simulink model "PWMverwerking"  (R2018b)
settings: Solver=VariableStepAuto  StartTime=0.0  StopTime=10.0  RelTol=1e-3
undefined symbols (not defined in the file or in its folder): sigbuilder_block
libraries: powerlib_meascontrol x2
settings Model: Creator=Roberto  LastModifiedBy=Roberto

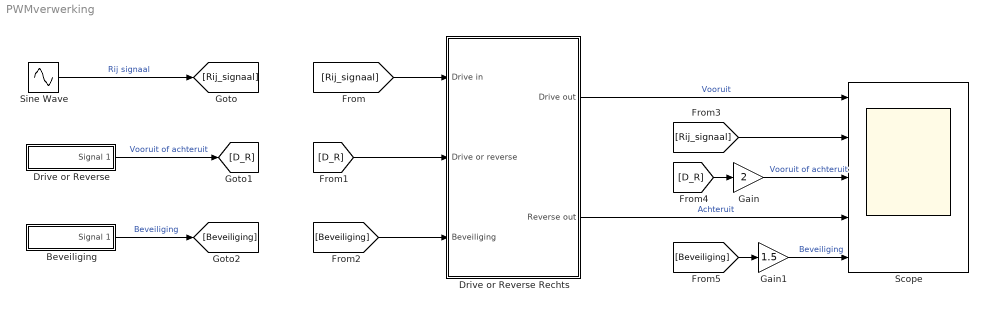
== system PWMverwerking ==
  Beveiliging : Subsystem  Tag=STV Subsys  LoadFcn=sigbuilder_block('load');  StartFcn=sigbuilder_block('start');  StopFcn=sigbuilder_block('stop');  ClipboardFcn=sigbuilder_block('clipboard');  mask(Sigbuilder block){tuvar=[0:10]}
      mask help: Simulink:masks:SigbuilderBlock_MD
      mask init:
      | if ~strcmp(get_param(bdroot(gcbh),'SimulationStatus'),'stopped') tuvar = sigbuilder_block('maskInit'); end
      settings: CopyFcn=sigbuilder_block('copy');  DeleteFcn=sigbuilder_block('delete');  ModelCloseFcn=sigbuilder_block('modelClose');  PreSaveFcn=sigbuilder_block('preSave');  PauseFcn=sigbuilder_block('pause');  ContinueFcn=sigbuilder_block('continue');  NameChangeFcn=sigbuilder_block('namechange');  OpenFcn=sigbuilder_block('open',[437.6 153 550.4 359.25 ]);  CloseFcn=sigbuilder_block('close');
      mask Display: plot(0, 0, 100, 100,[2, 2, 32, 32, 2], [68, 8, 8, 68, 68],[32, 2], [38, 38], [32, 19, 2],[53, 60, 44], [32, 17, 17, 2],[16, 16, 31, 31]);txt = getActiveGroup(gcbh);text(2, 100, txt,'verticalAlignment', 'top');
  Drive or Reverse : Subsystem  Tag=STV Subsys  LoadFcn=sigbuilder_block('load');  StartFcn=sigbuilder_block('start');  StopFcn=sigbuilder_block('stop');  ClipboardFcn=sigbuilder_block('clipboard');  mask(Sigbuilder block){tuvar=[0:10]}
      mask help: Simulink:masks:SigbuilderBlock_MD
      mask init:
      | if ~strcmp(get_param(bdroot(gcbh),'SimulationStatus'),'stopped') tuvar = sigbuilder_block('maskInit'); end
      settings: CopyFcn=sigbuilder_block('copy');  DeleteFcn=sigbuilder_block('delete');  ModelCloseFcn=sigbuilder_block('modelClose');  PreSaveFcn=sigbuilder_block('preSave');  PauseFcn=sigbuilder_block('pause');  ContinueFcn=sigbuilder_block('continue');  NameChangeFcn=sigbuilder_block('namechange');  OpenFcn=sigbuilder_block('open',[437.6 153 550.4 359.25 ]);  CloseFcn=sigbuilder_block('close');
      mask Display: plot(0, 0, 100, 100,[2, 2, 32, 32, 2], [68, 8, 8, 68, 68],[32, 2], [38, 38], [32, 19, 2],[53, 60, 44], [32, 17, 17, 2],[16, 16, 31, 31]);txt = getActiveGroup(gcbh);text(2, 100, txt,'verticalAlignment', 'top');
  Drive or Reverse Rechts : Subsystem
  Gain : Gain  Gain=2
  Gain1 : Gain  Gain=1.5
  Scope : Scope  NumInputPorts=5
  Sine Wave : Sin  SineType=Sample based  Samples=50000  SampleTime=1/10000
  wires:
  Drive or Reverse Rechts/1(Drive out) -> Scope/1  "Vooruit"
  Drive or Reverse Rechts/2(Reverse out) -> Scope/4  "Achteruit"
  [D_R] -> Drive or Reverse Rechts/2(Drive or reverse)
  [Beveiliging] -> Drive or Reverse Rechts/3(Beveiliging)
  [Rij_signaal] -> Drive or Reverse Rechts/1(Drive in)
  Drive or Reverse/1(Signal 1) -> [D_R]  "Vooruit of achteruit"
  Beveiliging/1(Signal 1) -> [Beveiliging]  "Beveiliging"
  [Rij_signaal] -> Scope/2
  [D_R] -> Gain/1
  [Beveiliging] -> Gain1/1
  Sine Wave/1 -> [Rij_signaal]  "Rij signaal"
  Gain/1 -> Scope/3  "Vooruit of achteruit"
  Gain1/1 -> Scope/5  "Beveiliging"

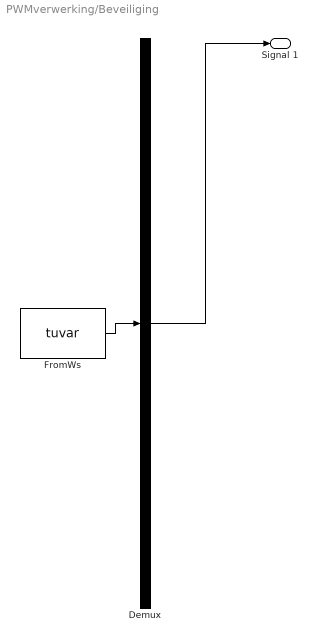
== system PWMverwerking/Beveiliging ==
  Demux : Demux  Tag=STV Demux  Outputs=1
  FromWs : FromWorkspace  Tag=STV FromWs  VariableName=tuvar  SampleTime=0
      SigBuilderData=|
      | common.afterFinalStr = 'Extrapolate'
      | common.sampleTime = 0
      | dataSet.timeRange = [0 10]
      | dataSet.name = 'Group 1'
      | sbobj.Groups.Name = 'Group 1'
      | sbobj.Groups.Signals.Name = 'Signal 1'
      | sbobj.Groups.Signals.XData = [0 1.5 1.5 2 2 4.5 4.5 5 5 8 8 9 9 9.6 10]
      | sbobj.Groups.Signals.YData = [0 0 1 1 0 0 1 1 0 0 1 1 0 0 0]
  Signal 1 : Outport  Tag=STV Outport
  wires:
  Demux/1 -> Signal 1/1
  FromWs/1 -> Demux/1

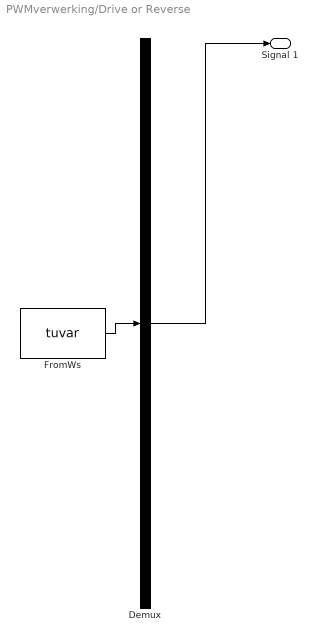
== system PWMverwerking/Drive or Reverse ==
  Demux : Demux  Tag=STV Demux  Outputs=1
  FromWs : FromWorkspace  Tag=STV FromWs  VariableName=tuvar  SampleTime=0
      SigBuilderData=|
      | common.afterFinalStr = 'Extrapolate'
      | common.sampleTime = 0
      | dataSet.timeRange = [0 10]
      | dataSet.name = 'Group 1'
      | sbobj.Groups.Name = 'Group 1'
      | sbobj.Groups.Signals.Name = 'Signal 1'
      | sbobj.Groups.Signals.XData = [0 3 3 7 7 9 9 9.6 10]
      | sbobj.Groups.Signals.YData = [1 1 0 0 1 1 0 0 0]
  Signal 1 : Outport  Tag=STV Outport
  wires:
  Demux/1 -> Signal 1/1
  FromWs/1 -> Demux/1

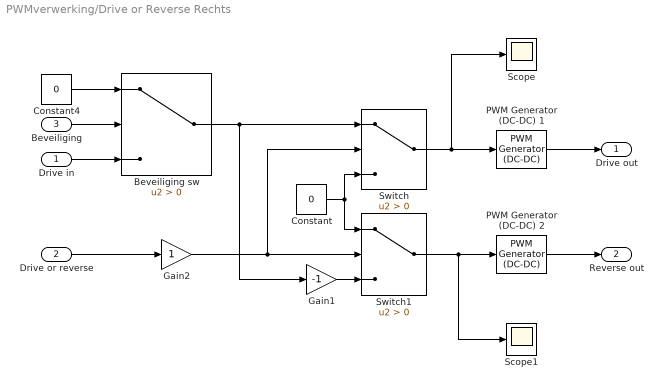
== system PWMverwerking/Drive or Reverse Rechts ==
  Drive in : Inport
  Drive or reverse : Inport  Port=2
  Beveiliging : Inport  Port=3
  Beveiliging sw : Switch  Criteria=u2 > Threshold
  Constant : Constant  Value=0
  Constant4 : Constant  Value=0
  Gain1 : Gain  Gain=-1
  Gain2 : Gain
  PWM Generator (DC-DC) 1 : powerlib_meascontrol/Pulse & Signal Generators/PWM Generator (DC-DC)  Fsw=20e3  Ts=1e-6
      settings: SourceProductName=Simscape Electrical
  PWM Generator (DC-DC) 2 : powerlib_meascontrol/Pulse & Signal Generators/PWM Generator (DC-DC)  Fsw=20e3  Ts=1e-6
      settings: SourceProductName=Simscape Electrical
  Scope : Scope
  Scope1 : Scope
  Switch : Switch  Criteria=u2 > Threshold
  Switch1 : Switch  Criteria=u2 > Threshold
  Drive out : Outport
  Reverse out : Outport  Port=2
  wires:
  Gain1/1 -> Switch1/3
  Switch1/1 -> Scope1/1, PWM Generator (DC-DC) 2/1
  Constant4/1 -> Beveiliging sw/1
  Constant/1 -> Switch1/1, Switch/3
  Beveiliging sw/1 -> Gain1/1, Switch/1
  Drive in/1 -> Beveiliging sw/3
  Beveiliging/1 -> Beveiliging sw/2
  Switch/1 -> PWM Generator (DC-DC) 1/1, Scope/1
  PWM Generator (DC-DC) 2/1 -> Reverse out/1
  Gain2/1 -> Switch/2, Switch1/2
  Drive or reverse/1 -> Gain2/1
  PWM Generator (DC-DC) 1/1 -> Drive out/1
